simulink model "simscape_custom_generator"  (R2014a)
settings: Solver=ode23t  StartTime=0.0  StopTime=0.1  MaxStep=1e-4  RelTol=1e-3
libraries: fl_lib x7, nesl_utility x5, pe_lib x4, ThreePhaseExamples_lib x1
Description:
  | Three-Phase Custom Synchronous Machine
  | 
  | This example shows a custom Simscape(TM) implementation of a Synchronous Machine (SM).
  | To view the SM source code, double-click on the Synchronous Machine block and then click on
  | the hyperlink 'Source code'.
  | 
  | This test circuit shows the SM being used as a generator, the field has constant voltage applied,
  | and the rotor is turned at a constant speed. The overall model has been initialized to start in
  | periodic steady state to supply the 500MW load.
  | 
  | 
  | Copyright 2008-2014 The MathWorks, Inc.
settings Model: Creator=MathWorks  LastModifiedBy=cosorio
settings DataIOCC: SaveOutput=off  SaveTime=off
settings DebuggingCC: UnderspecifiedInitializationDetection=Classic

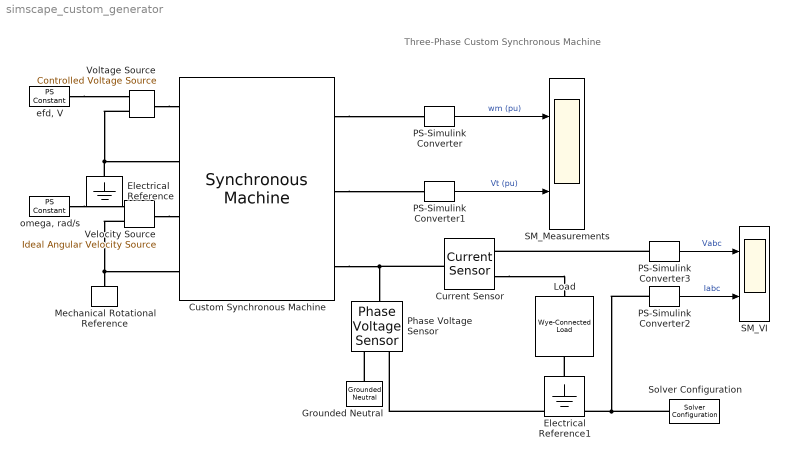
== system simscape_custom_generator ==
  note: Three-Phase Custom Synchronous Machine
  Current Sensor : pe_lib/Sensors/Current Sensor
  Custom Synchronous Machine : ThreePhaseExamples_lib/Synchronous Machine  SRated=555e6 V*A  VRated=24e3 V  FRated=60 Hz  nPolePairs=1  baseIfd=1300 A  Lad=1.66  Laq=1.61  Ll=0.15  Ra=0.003  Lfd=0.165  Rfd=0.0006  L1d=0.1713  R1d=0.0284  L1q=0.7252  R1q=0.00619  L2q=0.125  R2q=0.02368  angular_position_specify=on  angular_position_priority=High  angular_position=57.6913 rad  pu_psid_specify=on  pu_psid_priority=High  pu_psid=0.5359  pu_psiq_specify=on  pu_psiq_priority=High  pu_psiq=-0.8475  pu_psifd_specify=on  pu_psifd_priority=High  pu_psifd=0.8404  pu_psi1d_specify=on  pu_psi1d_priority=High  pu_psi1d=0.6501  pu_psi1q_specify=on  pu_psi1q_priority=High  pu_psi1q=-0.7752  pu_psi2q_specify=on  pu_psi2q_priority=High  pu_psi2q=-0.7752
  Electrical Reference : fl_lib/Electrical/Electrical Elements/Electrical Reference
  Electrical Reference1 : fl_lib/Electrical/Electrical Elements/Electrical Reference
  Grounded Neutral : pe_lib/Connections/Grounded Neutral
  Load : pe_lib/Passive Devices/Wye-Connected Load  parameterization=2  component_structure=1  component_structure_PQ=1  R=1 Ohm  L=0.001 H  C=1e-6 F  IL0=[ 0 0 0 ] A  VC0=[ 0 0 0 ] V  R_parasitic=1e-6 Ohm  G_parasitic=1e-6 1/Ohm  VRated=24e3 V  FRated=60 Hz  P=500e6 W  Qpos=100 V*A  Qneg=-100 V*A  Vmag0=2.4e+4 V  Vang0=0 deg  Freq0=60 Hz  R_parasitic_PQ=1e-6 Ohm  G_parasitic_PQ=1e-6 1/Ohm
  Mechanical Rotational Reference : fl_lib/Mechanical/Rotational Elements/Mechanical Rotational Reference
  PS-Simulink Converter{,1..3} (4 alike) : nesl_utility/PS-Simulink Converter  PhysicalDomain=network_engine_domain  SubClassName=ps_output  LeftPortType=input  RightPortType=output  PseudoPeriodic=off  Frequencies=[]  Unit=1  AffineConversion=off
  Phase Voltage Sensor : pe_lib/Sensors/Phase Voltage Sensor
  SM_Measurements : Scope  NumInputPorts=2
      settings: YMin=0~0  YMax=1.5~1.5  SaveName=SM_MeasData
  SM_VI : Scope  NumInputPorts=2
      settings: YMin=-25000~-25000  YMax=25000~25000  SaveName=SM_VIData
  Solver Configuration : nesl_utility/Solver Configuration  PhysicalDomain=network_engine_domain  SubClassName=solver  LeftPortType=input  RightPortType=generic  Accelerate=off  Tones=[]  Harmonics=[]  SimulateNoise=off  Profile=off  UseLocalSampling=off  EnableSwitchedLinearOptims=on  FrequencyDomain=off  UseCCode=off  RelTol=0.001  AbsTol=1e-06  MinStep=1e-09  ToWorkspace=off  DoDC=off  ResidualTolerance=1e-09  UseLocalSolver=off  LocalSolverChoice=NE_BACKWARD_EULER_ADVANCER  LocalSolverSampleTime=1e-4  DoFixedCost=off  MaxNonlinIter=3  MaxModeIter=2  LinearAlgebra=Sparse  DelaysMemoryBudget=1024  AutomaticFiltering=on  FilteringTimeConstant=0.001
  Velocity Source : fl_lib/Mechanical/Mechanical Sources/Ideal Angular Velocity Source
  Voltage Source : fl_lib/Electrical/Electrical Sources/Controlled Voltage Source
  "efd, V" : fl_lib/Physical Signals/Sources/PS Constant  constant=177.93
  "omega, rad/s" : fl_lib/Physical Signals/Sources/PS Constant  constant=2*pi*60
  wires:
  PS-Simulink Converter/1 -> SM_Measurements/1  "wm (pu)"
  PS-Simulink Converter1/1 -> SM_Measurements/2  "Vt (pu)"
  PS-Simulink Converter3/1 -> SM_VI/1  "Vabc"
  PS-Simulink Converter2/1 -> SM_VI/2  "Iabc"
  connections:
  Voltage Source/LConn1 -- Custom Synchronous Machine/LConn1
  Voltage Source/RConn2 -- Custom Synchronous Machine/LConn2 -- Electrical Reference/LConn1
  Velocity Source/LConn1 -- Custom Synchronous Machine/LConn3
  Velocity Source/RConn2 -- Custom Synchronous Machine/LConn4 -- Mechanical Rotational Reference/LConn1
  Custom Synchronous Machine/RConn1 -- PS-Simulink Converter/LConn1
  Custom Synchronous Machine/RConn2 -- PS-Simulink Converter1/LConn1
  "efd, V"/RConn1 -- Voltage Source/RConn1
  "omega, rad/s"/RConn1 -- Velocity Source/RConn1
  Custom Synchronous Machine/RConn3 -- Current Sensor/LConn1 -- Phase Voltage Sensor/LConn1
  Electrical Reference1/LConn1 -- Load/RConn1
  Grounded Neutral/LConn1 -- Phase Voltage Sensor/RConn2
  PS-Simulink Converter2/LConn1 -- Solver Configuration/RConn1 -- Phase Voltage Sensor/RConn1
  Current Sensor/RConn2 -- Load/LConn1
  PS-Simulink Converter3/LConn1 -- Current Sensor/RConn1
